simulink model "validar_espacio_estado_Objeto_simulink"  (R2017b)
settings: Solver=VariableStepAuto  StartTime=0.0  StopTime=15  RelTol=1e-3
settings Model: Creator=xmax1  LastModifiedBy=xmax1

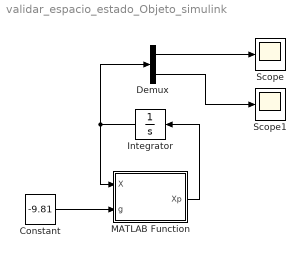
== system validar_espacio_estado_Objeto_simulink ==
  Constant : Constant  Value=-9.81
  Demux : Demux  Outputs=2
  Integrator : Integrator  InitialCondition=[0 ; 100]
  MATLAB Function : MATLAB Function  TreatAsAtomicUnit=on
  Scope : Scope
  Scope1 : Scope
  wires:
  MATLAB Function/1(Xp) -> Integrator/1
  Integrator/1 -> Demux/1, MATLAB Function/1(X)
  Demux/1 -> Scope/1
  Constant/1 -> MATLAB Function/2(g)
  Demux/2 -> Scope1/1

== matlab function validar_espacio_estado_Objeto_simulink/MATLAB Function ==
  data: X input; Xp output; g input
function Xp = Objeto(X, g)

D = 1 * 10^-1;
m = 1;

A = [0, 1 ; 0, -D/m];
B = [0 ; 1];

Xp = A*X + B*g;
